simulink model "Vision_Controller_Algorithm_soln"  (R2018a)
settings: Solver=FixedStepAuto  StartTime=0.0  StopTime=inf  RelTol=1e-3
PreLoadFcn:
  | initParams;
settings Model: Creator=cdsouza  LastModifiedBy=scastro
settings DataIOCC: SaveOutput=off  SaveTime=off
settings OptimizationCC: DefaultParameterBehavior=Inlined  EnhancedBackFolding=on  PassReuseOutputArgsAs=Individual arguments  OptimizeBlockOrder=speed  DifferentSizesBufferReuse=on  OptimizationCustomize=off
settings DebuggingCC: ParameterTunabilityLossMsg=error
settings SFSimCC: MATLABDynamicMemAlloc=off
settings RTWCC: SystemTargetFile=ert.tlc  TemplateMakefile=ert_default_tmf  GenerateReport=on  IncludeHyperlinkInReport=on  LaunchReport=on  GenerateTraceInfo=on  GenerateTraceReport=on  GenerateTraceReportSl=on  GenerateTraceReportSf=on  GenerateTraceReportEml=on
settings CodeAppCC: ForceParamTrailComments=on  IgnoreCustomStorageClasses=off  OperatorAnnotations=on  SimulinkDataObjDesc=on  SFDataObjDesc=on  InsertBlockDesc=on
settings ERTTargetCC: TargetLangStandard=C99 (ISO)  GenerateSampleERTMain=on  SupportVariableSizeSignals=on  InlinedParameterPlacement=NonHierarchical  ERTCustomFileTemplate=example_file_process.tlc

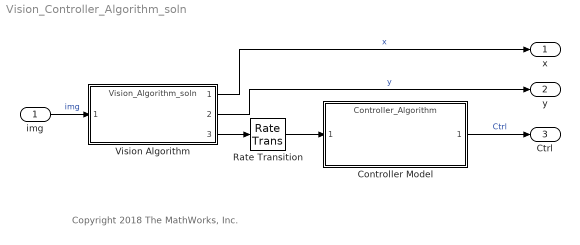
== system Vision_Controller_Algorithm_soln ==
  note: Copyright 2018 The MathWorks, Inc.
  img : Inport  OutDataTypeStr=uint8  PortDimensions=[240 320 3]  SampleTime=[0.050000000000000003,0]
  Controller Model : ModelReference  ModelNameDialog=Controller_Algorithm.slx  SimulationMode=Normal  ModelReferenceVersion=1.21
  Rate Transition : RateTransition
  Vision Algorithm : ModelReference  ModelNameDialog=Vision_Algorithm_soln  SimulationMode=Normal  ModelReferenceVersion=1.36
  x : Outport  OutDataTypeStr=double  PortDimensions=1  SampleTime=[0.050000000000000003,0]
  y : Outport  Port=2  OutDataTypeStr=double  PortDimensions=1  SampleTime=[0.050000000000000003,0]
  Ctrl : Outport  Port=3  OutDataTypeStr=double  PortDimensions=1  SampleTime=[0.01,0]
  wires:
  Controller Model/1 -> Ctrl/1  "Ctrl"
  Vision Algorithm/3 -> Rate Transition/1
  img/1 -> Vision Algorithm/1  "img"
  Rate Transition/1 -> Controller Model/1
  Vision Algorithm/1 -> x/1  "x"
  Vision Algorithm/2 -> y/1  "y"
